simulink model "simulink_experiments_LQ_obs"  (R2019b)
settings: Solver=ode1  StartTime=0.0  StopTime=inf  FixedStep=0.002  RelTol=1e-3  EnableMultiTasking=on
PostLoadFcn:
  | qc_set_target_type(getConfigSet(bdroot, 'QUARC Default Target Configuration'));
undefined symbols (not defined in the file): Ao, Bo, HIL, Klqi_int, Klqi_state, qc_get_step_size
libraries: quarc_library x4
settings Model: SimulationMode=external  ExtModeTrigDuration=5000  Creator=CFulford  LastModifiedBy=Samsung
settings SolverCC: PositivePriorityOrder=on
settings DataIOCC: LimitDataPoints=on  SaveFormat=Array  SignalLoggingSaveFormat=ModelDataLogs  ReturnWorkspaceOutputs=off
settings OptimizationCC: ExpressionDepthLimit=2147483647  InitFltsAndDblsToZero=on  LifeSpan=inf
settings DebuggingCC: SaveWithParameterizedLinksMsg=none  UnderspecifiedInitializationDetection=Classic  MergeDetectMultiDrivingBlocksExec=none  SolverPrmCheckMsg=warning  MultiTaskDSMMsg=warning  MultiTaskCondExecSysMsg=none  FcnCallInpInsideContextMsg=warning  StateNameClashWarn=warning  SFUnexpectedBacktrackingDiag=warning  SFNoUnconditionalDefaultTransitionDiag=warning  SFExecutionAtInitializationDiag=none  ArithmeticOperatorsInVariantConditions=warning
settings HardwareCC: ProdBitPerPointer=32  ProdBitPerSizeT=32  ProdBitPerPtrDiffT=32  ProdLargestAtomicFloat=None  ProdIntDivRoundTo=Undefined  ProdEndianess=Unspecified  ProdWordSize=32  ProdHWDeviceType=32-bit Generic
settings ModelReferenceCC: PropagateSignalLabelsOutOfModel=off
settings SFSimCC: SimUseLocalCustomCode=off  CustomCodeUndefinedFunction=UseInterfaceOnly
settings RTWCC: Description=QUARC Win64 Target  SystemTargetFile=quarc_win64.tlc  TemplateMakefile=quarc_default_tmf  RTWUseLocalCustomCode=off
settings CodeAppCC: StateflowObjectComments=on
settings STFCustomTargetCC: TargetPreCompLibLocation=C:\PROGRA~3\QUARC\lib\2019b\win64\release  ConcurrentExecutionCompliant=on  GeneratePreprocessorConditionals=Disable all  CombineOutputUpdateFcns=on  CPPClassGenCompliant=on  SystemTargetFile=quarc_win64.tlc
settings GRTTargetCC: TargetPreCompLibLocation=C:\PROGRA~3\QUARC\lib\2019b\win64\release  TargetLangStandard=C89/C90 (ANSI)  ParMdlRefBuildCompliant=off  CompOptLevelCompliant=off  GeneratePreprocessorConditionals=Disable all  MatFileLogging=off  UseToolchainInfoCompliant=off  ExtMode=on  ExtModeMexFile=quarc_comm
settings ConfigComp: CovMetricSettings=dw  CovHtmlReporting=on  CovSaveCumulativeToWorkspaceVar=on  CovSaveSingleToWorkspaceVar=on  CovExternalEMLEnable=off  CovSFcnEnable=off

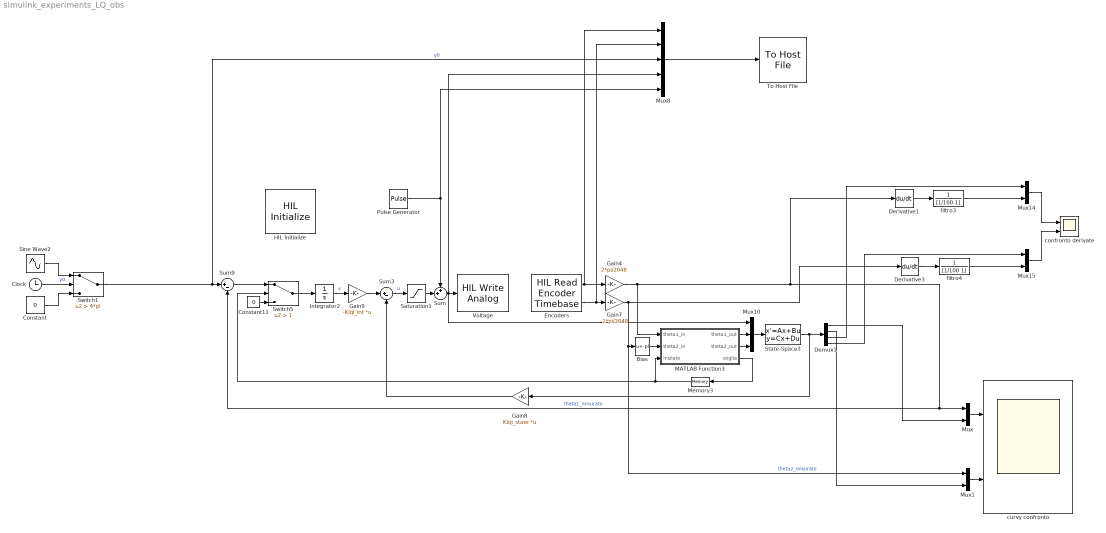
== system simulink_experiments_LQ_obs ==
  Bias : Bias  Bias=-pi
  Clock : Clock
  Constant : Constant  Value=0
  Constant11 : Constant  Value=0
  Demux1 : Demux
  Derivative1 : Derivative
  Derivative3 : Derivative
  Encoders : quarc_library/Data Acquisition/Generic/Timebases/HIL Read Encoder Timebase  object_name=HIL-1  clock=0  channels=[0:1]  samples_in_buffer=max(ceil(1/qc_get_step_size), 1)  active=on  vector_output=off  data_type_mode=Inherit via back propagation  data_type=double
  Gain4 : Gain  Gain=2*pi/2048
  Gain7 : Gain  Gain=-2*pi/2048
  Gain8 : Gain  Gain=Klqi_state  Multiplication=Matrix(K*u)
  Gain9 : Gain  Gain=-Klqi_int  Multiplication=Matrix(K*u)
  HIL Initialize : quarc_library/Data Acquisition/Generic/Configuration/HIL Initialize  Priority=-99  object_name=HIL-1  board_type=qube_servo2_usb  board_number=0  board_options=""  exclusive=off  active=off  hardware_clocks=[0]  clock_modes=[]  initial_clock_frequencies=[]  set_clock_params_at_start=off  set_clock_params_at_switch_in=off  set_clock_frequencies_at_start=off  set_clock_frequencies_at_switch_in=off  analog_input_channels=[0]  analog_input_configurations=[]  analog_input_maximums=3  analog_input_minimums=-3  set_analog_input_params_at_start=off  set_analog_input_params_at_switch_in=off  analog_output_channels=[0]  analog_output_maximums=15  analog_output_minimums=-15  initial_analog_outputs=[0]  final_analog_outputs=[0]  watchdog_analog_outputs=0  set_analog_output_params_at_start=off  set_analog_output_params_at_switch_in=off  set_analog_outputs_at_start=on  set_analog_outputs_at_switch_in=off  set_analog_outputs_at_terminate=on  set_analog_outputs_at_switch_out=off  set_analog_outputs_on_watchdog=on  digital_input_channels=[]  digital_output_channels=[0]  digital_output_configuration=[]  initial_digital_outputs=[1]  final_digital_outputs=[0]  watchdog_digital_outputs=[0]  set_digital_output_params_at_start=off  set_digital_output_params_at_switch_in=off  set_digital_outputs_at_start=on  set_digital_outputs_at_switch_in=off  set_digital_outputs_at_terminate=on  set_digital_outputs_at_switch_out=off  set_digital_outputs_on_watchdog=on  encoder_channels=[0:1]  quadrature=[4]  encoder_filter_frequency=[]  initial_encoder_counts=[0]  set_encoder_params_at_start=off  set_encoder_params_at_switch_in=off  set_encoder_counts_at_start=on  set_encoder_counts_at_switch_in=off  pwm_channels=[]  pwm_modes=[]  pwm_frequency=[]  pwm_configuration=[]  pwm_alignment=[]  pwm_polarity=[]  pwm_leading_deadband=[]  pwm_trailing_deadband=[]  initial_pwm_outputs=[]  final_pwm_outputs=[]  watchdog_pwm_outputs=[]  set_pwm_params_at_start=off  set_pwm_params_at_switch_in=off  set_pwm_outputs_at_start=off  set_pwm_outputs_at_switch_in=off  set_pwm_outputs_at_terminate=off  set_pwm_outputs_at_switch_out=off  set_pwm_outputs_on_watchdog=off  other_output_channels=[11000:11002]  initial_other_outputs=[0 1 0]  final_other_outputs=[1 0 0]  watchdog_other_outputs=[0 0 1]  set_other_outputs_at_start=on  set_other_outputs_at_switch_in=off  set_other_outputs_at_terminate=on  set_other_outputs_at_switch_out=off  set_other_outputs_on_watchdog=on
  Integrator2 : Integrator
  MATLAB Function3 : MATLAB Function  TreatAsAtomicUnit=on
  Memory3 : Memory
  Mux{,1,14..15} (4 alike) : Mux  Inputs=2
  Mux10 : Mux  Inputs=3
  Mux8 : Mux  Inputs=5
  Pulse Generator : DiscretePulseGenerator  PulseType=Time based  Amplitude=0.8  Period=10
  Saturation1 : Saturate  UpperLimit=10  LowerLimit=-10
  Sine Wave2 : Sin  SampleTime=0
  State-Space3 : StateSpace  A=Ao  B=Bo  C=eye(4)  D=zeros(4,3)  InitialCondition=0
  Sum : Sum  Inputs=++|
  Sum3 : Sum  Inputs=|+-
  Sum9 : Sum  Inputs=|+-
  Switch1 : Switch  Criteria=u2 > Threshold  Threshold=4*pi
  Switch5 : Switch  Criteria=u2 > Threshold  Threshold=1
  To Host File : quarc_library/Sinks/To Host/To Host File  file_name=data_%{date}_%{time}.mat  variable_name=data_%{date}_%{time}  decimation=1  sample_time=-1  file_format=MAT-file v.5  options=No header or footer  append=off  final_file_name=data_17-May-2024_10-33-04.mat  bitrate=2000000
  Voltage : quarc_library/Data Acquisition/Generic/Immediate I//O/HIL Write Analog  object_name=HIL-1  channels=0  sample_time=-1  active=off  vector_input=off
  "confronto derivate " : Scope  NumInputPorts=2
  curvy confronto : Scope  NumInputPorts=2
  filtro3 : TransferFcn  Denominator=[1/100 1]
  filtro4 : TransferFcn  Denominator=[1/100 1]
  wires:
  Mux8/1 -> To Host File/1
  Gain4/1 -> MATLAB Function3/1(theta1_in), Derivative1/1, Sum9/2, Mux/1  "theta1_misurato"
  Encoders/1 -> Gain4/1, Mux8/1
  Mux10/1 -> State-Space3/1
  Derivative3/1 -> filtro4/1
  Mux14/1 -> "confronto derivate "/1
  Gain9/1 -> Sum3/1
  Integrator2/1 -> Gain9/1  "v"
  Derivative1/1 -> filtro3/1
  filtro4/1 -> Mux15/2
  Switch5/1 -> Integrator2/1
  Sum9/1 -> Switch5/1
  Memory3/1 -> MATLAB Function3/3(iniziato), Switch5/2
  MATLAB Function3/2(theta2_out) -> Mux10/3
  Gain8/1 -> Sum3/2
  MATLAB Function3/1(theta1_out) -> Mux10/2
  Gain7/1 -> Mux1/1, Bias/1, Derivative3/1  "theta2_misurato"
  Bias/1 -> MATLAB Function3/2(theta2_in)
  Constant11/1 -> Switch5/3
  MATLAB Function3/3(soglia) -> Memory3/1
  State-Space3/1 -> Demux1/1, Gain8/1
  filtro3/1 -> Mux14/2
  Encoders/2 -> Mux8/2, Gain7/1
  Sum3/1 -> Saturation1/1  "u"
  Mux15/1 -> "confronto derivate "/2
  Switch1/1 -> Mux8/3, Sum9/1  "y0"
  Saturation1/1 -> Sum/2
  Sum/1 -> Mux8/4, Mux10/1, Voltage/1
  Pulse Generator/1 -> Mux8/5, Sum/1
  Clock/1 -> Switch1/2
  Constant/1 -> Switch1/3
  Sine Wave2/1 -> Switch1/1  "y0"
  Demux1/4 -> Mux15/1
  Demux1/3 -> Mux14/1
  Demux1/1 -> Mux/2
  Demux1/2 -> Mux1/2
  Mux1/1 -> curvy confronto/2
  Mux/1 -> curvy confronto/1

== matlab function simulink_experiments_LQ_obs/MATLAB Function3 ==
  data: theta1_in input; theta1_out output; theta2_out output; theta2_in input; iniziato input double; soglia output
function [theta1_out, theta2_out, soglia] = fcn(theta1_in, theta2_in, iniziato)
if theta2_in >= 0.01
    theta1_out = theta1_in;
    theta2_out = theta2_in;
    soglia = 2; 
elseif iniziato >1
    theta1_out = theta1_in;
    theta2_out = theta2_in;
    soglia = 2;
else
    soglia = 0;
    theta1_out = 0;
    theta2_out = 0;
end
end
